simulink model "Resistor_CurrentBased"  (R2020b)
settings: Solver=VariableStepAuto  StartTime=0.0  StopTime=10.0  RelTol=1e-3
libraries: Lib_PB_BuckConv_TMATS x1
settings Model: Creator=mebell  LastModifiedBy=nbutler2
settings DataIOCC: ReturnWorkspaceOutputs=off
settings DebuggingCC: ArithmeticOperatorsInVariantConditions=warning
settings SFSimCC: SimUseLocalCustomCode=off  CustomCodeUndefinedFunction=UseInterfaceOnly
settings RTWCC: RTWUseLocalCustomCode=off

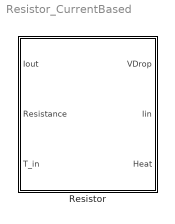
== system Resistor_CurrentBased ==
  Resistor : Subsystem  mask{TempIn=Celsius}
      mask prompts: TempIn "Input Units"
      mask init:
      | %Get current block name
      | block = gcb;
      | 
      | %Block under the mask(T_in inport and outport)
      | block2 = [block '/T_in'];
      | 
      | %Set T_in unit parameter to correct unit.
      | switch TempIn
      |     case 1 
      |         set_param(block2,'Unit','degF');
      |     case 2
      |         set_param(block2,'Unit','degC');
      |     case 3
      |         set_param(block2,'Unit','degR');
      |     case 4
      |         set_param(block2,'Unit','K');
      | end
      mask TypeOptions TempIn: Fahrenheit | Celsius | Rankine | Kelvin
      mask DialogControl Container4 Prompt: Parameters
      mask DialogControl Container8 Prompt: Temperature Units
      mask Display:
      | switch TempIn
      |     case 1
      |         port_label('input', 3, 'T_in (F)');
      |     case 2
      |         port_label('input', 3, 'T_in (C)');
      |     case 3
      |         port_label('input', 3, 'T_in (Ra)');
      |     case 4
      |         port_label('input', 3, 'T_in (K)');
      | end
      | 
      | 
      | port_label('input', 1, 'Idemand');
      | port_label('input', 2, 'Resistance');
      | 
      | 
      | port_label('output', 1, 'VDrop');
      | port_label('output', 2, 'Idemanded');
      | port_label('output', 3, 'Heat');

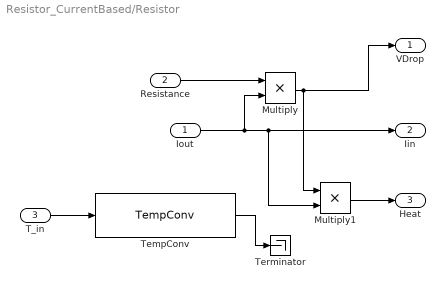
== system Resistor_CurrentBased/Resistor ==
  Iout : Inport
  Resistance : Inport  Port=2
  T_in : Inport  Port=3  Unit=degC
  Multiply : Product
  Multiply1 : Product
  TempConv : Lib_PB_BuckConv_TMATS/Buck Converter/TempConv 
  Terminator : Terminator
  VDrop : Outport  VectorParamsAs1DForOutWhenUnconnected=off
  Iin : Outport  Port=2  VectorParamsAs1DForOutWhenUnconnected=off
  Heat : Outport  Port=3  VectorParamsAs1DForOutWhenUnconnected=off
  wires:
  Iout/1 -> Multiply/2, Multiply1/2, Iin/1
  Multiply/1 -> VDrop/1, Multiply1/1
  Resistance/1 -> Multiply/1
  Multiply1/1 -> Heat/1
  T_in/1 -> TempConv/1
  TempConv/1 -> Terminator/1
